simulink model "howitsdone"  (R2022a)
settings: Solver=FixedStepAuto  StartTime=0.0  StopTime=3  FixedStep=10e-5  RelTol=1e-3
values from neighbouring files (symbols this model uses):
  den = [4e-05 0.022 1 0]    [K.mat]    (also in K1.mat)
settings Model: Creator=mikol  LastModifiedBy=mikol

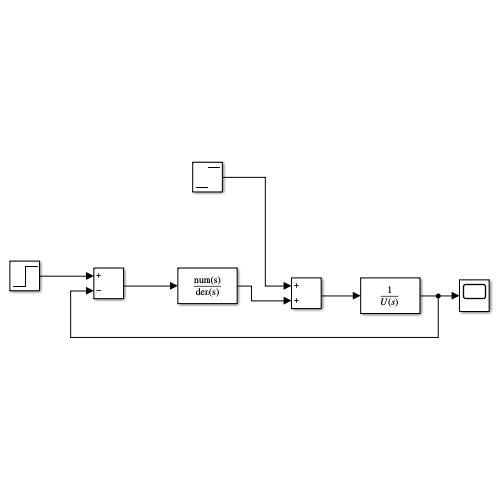
[thumbnail: Simulink's stored preview of the top-level diagram]
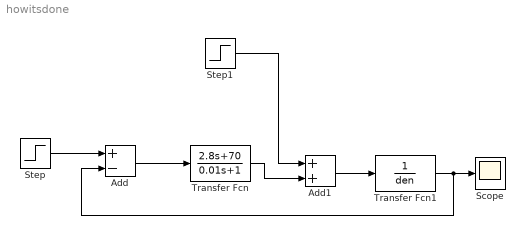
== system howitsdone ==
  Add : Sum  Inputs=+-
  Add1 : Sum
  Scope : Scope
  Step : Step  SampleTime=0
  Step1 : Step  SampleTime=0
  Transfer Fcn : TransferFcn  Numerator=[2.8 70]  Denominator=[0.01 1]
  Transfer Fcn1 : TransferFcn  Numerator=1  Denominator=den
  wires:
  Step1/1 -> Add1/1
  Transfer Fcn/1 -> Add1/2
  Add1/1 -> Transfer Fcn1/1
  Add/1 -> Transfer Fcn/1
  Step/1 -> Add/1
  Transfer Fcn1/1 -> Add/2, Scope/1
